simulink model "Final_Model"  (R2022b)
settings: Solver=VariableStepAuto  StartTime=0.0  StopTime=360  RelTol=1e-3  AbsTol=1e-3
InitFcn:
  | RT_env = 30; % [degC] External environment temperature
  | RH_env = 0.5; % External environment relative humidity
  | 
  | RH_house_init = 0.5; % Initial house relative humidity
  | 
  | tube_D = 0.02; % [m] Refrigerant tube diameter
  | duct_W = 0.4; % [m] Air duct width
  | 
  | house_L = 20; % [m] House length
  | house_W = 10; % [m] House width
  | house_H = 6; % [m] House height
  | roof_pitch = 40; % [deg] Roof pitch
  | A_I
  | A_IV
  | A_VIII
  | A_V
  | B_II
  | A_II
  | A_VI
undefined symbols (not defined in the file or in its folder): alpha_h_ratio, area_furniture, area_roof, area_wall_exterior, area_window, cp_furniture, cp_roof, cp_wall_exterior, cp_window, hc_furniture_interior, hc_roof_exterior, hc_roof_interior, hc_wall_exterior, hc_wall_interior, hc_window_exterior, hc_window_interior, k_roof, k_wall, k_window, l_roof, mass_furniture, no_motors, no_occupants, pitch_roof, Q_infiltration, Q_latent_occupant_skin, Q_lights, Q_occupant, rho_roof, rho_wall, rho_window, SC, sigbuilder_block, T_house_init, T_init_furniture, T_set, thicnkess_roof, thicnkess_wall_exterior, thicnkess_window, U_roof, U_wall, U_window, w_roof
libraries: fl_lib x89, nesl_utility x24, SimscapeFluids_lib x15, simulink_extras x4
(part 2 of 4)

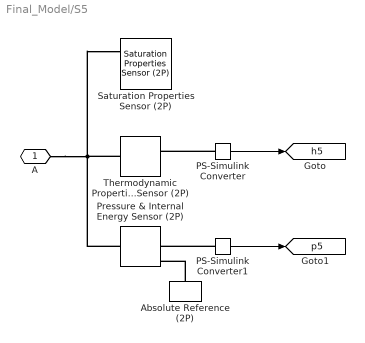
== system Final_Model/S5 ==
  Absolute Reference (2P) : fl_lib/Two-Phase Fluid/Elements/Absolute Reference (2P)
  PS-Simulink Converter : nesl_utility/PS-Simulink Converter  PhysicalDomain=network_engine_domain  SubClassName=ps_output  LeftPortType=input  RightPortType=output  PseudoPeriodic=off  Frequencies=[]  VectorFormat=inherit  Unit=kJ/kg  AffineConversion=off
  PS-Simulink Converter1 : nesl_utility/PS-Simulink Converter  PhysicalDomain=network_engine_domain  SubClassName=ps_output  LeftPortType=input  RightPortType=output  PseudoPeriodic=off  Frequencies=[]  VectorFormat=inherit  Unit=MPa  AffineConversion=off
  Pressure & Internal Energy Sensor (2P) : fl_lib/Two-Phase Fluid/Sensors/Pressure & Internal Energy Sensor (2P)
      settings: InternalSimscapePortConfiguration="{\"Bottom\":[],\"Left\":[{\"id\":\"A\",\"label\":\"A\",\"type\":\"foundation.two_phase_fluid.two_phase_fluid\"}],\"Right\":[{\"id\":\"B\",\"label\":\"B\",\"type\":\"foundation.two_phase_fluid.two_phase_fluid\"},{\"id\":\"P\",\"label\":\"P\",\"type\":\"output\"},{\"id\":\"U\",\"label\":\"U\",\"type\":\"output\"}],\"Top\":[]}"
  Saturation Properties Sensor (2P) : fl_lib/Two-Phase Fluid/Sensors/Saturation Properties Sensor (2P)  pressure_measure=simscape.enum.onoff.off  pressure_check=simscape.enum.assert.action.error  energy_measure=foundation.enum.EnergyMeasurement.SaturatedEnthalpy  density_measure=foundation.enum.DensityMeasurement.Off
      settings: InternalSimscapePortConfiguration="{\"Bottom\":[],\"Left\":[{\"id\":\"A\",\"label\":\"A\",\"type\":\"foundation.two_phase_fluid.two_phase_fluid\"}],\"Right\":[{\"id\":\"T_sat_liq\",\"label\":\"TL\",\"type\":\"output\"},{\"id\":\"T_sat_vap\",\"label\":\"TV\",\"type\":\"output\"}],\"Top\":[{\"id\":\"h_sat_liq\",\"label\":\"HL\",\"type\":\"output\"},{\"id\":\"h_sat_vap\",\"label\":\"HV\",\"type\":\"output\"}]}"
  Thermodynamic Properties Sensor (2P) : fl_lib/Two-Phase Fluid/Sensors/Thermodynamic Properties Sensor (2P)
      settings: InternalSimscapePortConfiguration="{\"Bottom\":[],\"Left\":[{\"id\":\"A\",\"label\":\"A\",\"type\":\"foundation.two_phase_fluid.two_phase_fluid\"}],\"Right\":[{\"id\":\"T\",\"label\":\"T\",\"type\":\"output\"},{\"id\":\"H\",\"label\":\"h\",\"type\":\"output\"},{\"id\":\"V\",\"label\":\"v\",\"type\":\"output\"},{\"id\":\"S\",\"label\":\"s\",\"type\":\"output\"}],\"Top\":[]}"
  A : PMIOPort  Side=Left
  tag scope: h5=global, p5=global
  wires:
  PS-Simulink Converter/1 -> [h5]
  PS-Simulink Converter1/1 -> [p5]
  connections:
  Pressure & Internal Energy Sensor (2P)/LConn1 -- Saturation Properties Sensor (2P)/LConn1 -- Thermodynamic Properties Sensor (2P)/LConn1 -- A/RConn1
  Absolute Reference (2P)/LConn1 -- Pressure & Internal Energy Sensor (2P)/RConn1
  PS-Simulink Converter/LConn1 -- Thermodynamic Properties Sensor (2P)/RConn2
  PS-Simulink Converter1/LConn1 -- Pressure & Internal Energy Sensor (2P)/RConn2

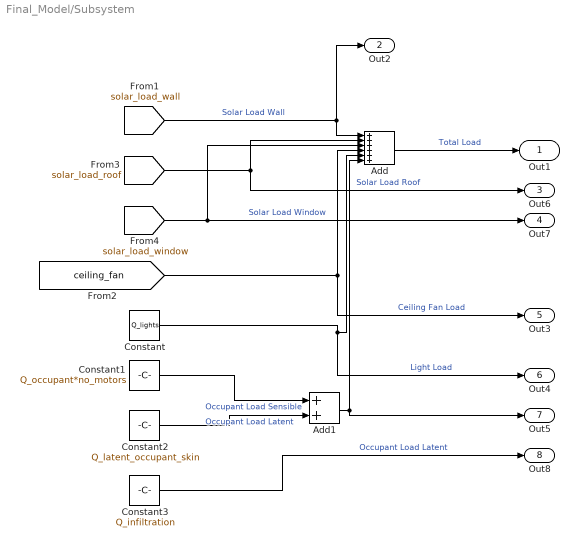
== system Final_Model/Subsystem ==
  Add : Sum  Inputs=++++++
  Add1 : Sum
  Constant : Constant  Value=Q_lights
  Constant1 : Constant  Value=Q_occupant*no_motors
  Constant2 : Constant  Value=Q_latent_occupant_skin
  Constant3 : Constant  Value=Q_infiltration
  Out1 : Outport
  Out2 : Outport  Port=2
  Out6 : Outport  Port=3
  Out7 : Outport  Port=4
  Out3 : Outport  Port=5
  Out4 : Outport  Port=6
  Out5 : Outport  Port=7
  Out8 : Outport  Port=8
  wires:
  Constant/1 -> Out4/1, Add/5  "Light Load"
  [ceiling_fan] -> Out3/1, Add/4  "Ceiling Fan Load"
  [solar_load_wall] -> Add/1, Out2/1  "Solar Load Wall"
  Add/1 -> Out1/1  "Total Load"
  [solar_load_roof] -> Add/2, Out6/1  "Solar Load Roof"
  [solar_load_window] -> Out7/1, Add/3  "Solar Load Window"
  Constant1/1 -> Add1/1  "Occupant Load Sensible"
  Constant2/1 -> Add1/2  "Occupant Load Latent"
  Add1/1 -> Add/6, Out5/1
  Constant3/1 -> Out8/1  "Occupant Load Latent"
